simulink model "Final_Project"  (R2021b)
settings: Solver=VariableStepAuto  StartTime=0.0  StopTime=10.0  RelTol=1e-3
undefined symbols (not defined in the file or in its folder): A, Aobs, B, Bobs, C, Cobs, Cobs1, Continuous, D, Dobs, K, N2, r0, Time
libraries: ctrlSharedLib x1, slpidlib x1
settings Model: Creator=AzamaoZ  LastModifiedBy=AzamaoZ
settings DataIOCC: ExternalInput=getinputstruct(op_trim1)  InitialState=getstatestruct(op_trim1)  LoadExternalInput=on  LoadInitialState=on

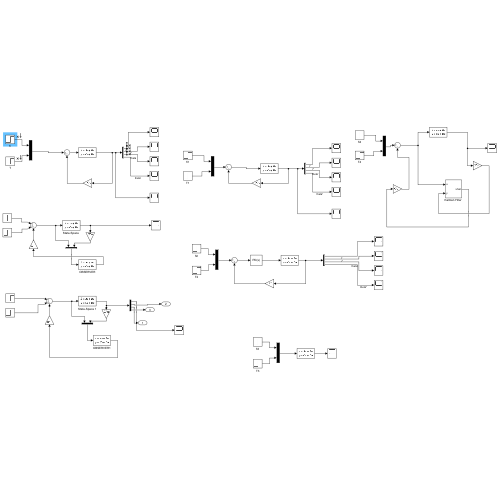
[thumbnail: Simulink's stored preview of the top-level diagram]
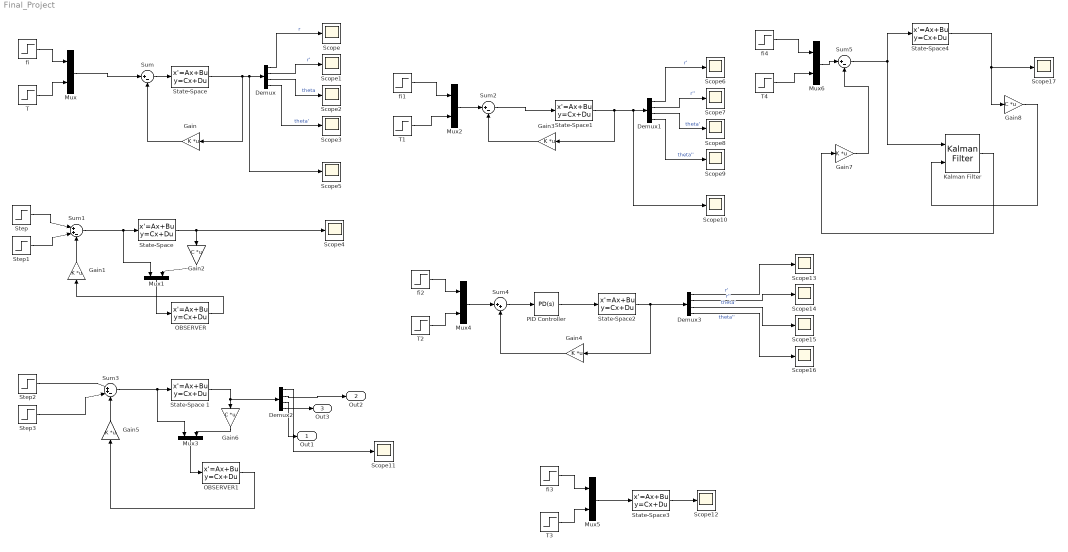
== system Final_Project ==
  Demux{,1..3} (4 alike) : Demux
  Gain{,1,3..5,7} (6 alike) : Gain  Gain=K  Multiplication=Matrix(K*u)
  Gain2 : Gain  Gain=C  Multiplication=Matrix(K*u)
  Gain6 : Gain  Gain=C  Multiplication=Matrix(K*u)
  Gain8 : Gain  Gain=C  Multiplication=Matrix(K*u)
  "Kalman Filter " : ctrlSharedLib/Kalman Filter  TimeDomain=Continuous-Time  UseCurrentEstimator=on  ModelSource=Individual A, B, C, D matrices  ModelSourceVariable=ss(0.95,1,1,0,1)  A=A  B=B  C=C  D=D  NumberOfStates=1  NumberOfInputs=1  NumberOfOutputs=1  InitialEstimateSource=Dialog  X0=10  P0=10  UseK=off  UseGH=off  NumberOfProcessNoiseInputs=1  G=1  TimeInvariantG=on  H=0  TimeInvariantH=on  Q=Q2  TimeInvariantQ=on  R=200  TimeInvariantR=on  N=N2  TimeInvariantN=on  AddInputPort=on  AddEnablePort=off  OutputEstimatedY=off  OutputP=off  Ts=-1
  Mux{,1..6} (7 alike) : Mux  Inputs=2
  OBSERVER : StateSpace  A=Aobs  B=Bobs  C=C  D=Dobs  InitialCondition=0
  OBSERVER1 : StateSpace  A=Aobs  B=Bobs  C=Cobs  D=Dobs  InitialCondition=0
  PID Controller : slpidlib/PID Controller  Controller=PD  Form=Parallel  TimeDomain=Continuous-time  UseExternalTs=off  SampleTime=-1  IntegratorMethod=Forward Euler  FilterMethod=Forward Euler  ControllerParametersSource=internal  P=0.02  I=1  D=0.01  UseFilter=on  N=100  TunerSelectOption=Frequency Response Based  InitialConditionSource=internal  InitialConditionForIntegrator=0  InitialConditionForFilter=0  DifferentiatorICPrevScaledInput=0  ExternalReset=none  TrackingMode=off  Kt=1  LimitOutput=off  SatLimitsSource=internal  UpperSaturationLimit=inf  LowerSaturationLimit=-inf  LinearizeAsGain=on  AntiWindupMode=none  Kb=1  POutMin=[]  POutMax=[]  IOutMin=[]  IOutMax=[]  DOutMin=[]  DOutMax=[]  NOutMin=[]  NOutMax=[]  SumOutMin=[]  SumOutMax=[]  SaturationOutMin=[]  SaturationOutMax=[]  PParamMin=[]  PParamMax=[]  IParamMin=[]  IParamMax=[]  DParamMin=[]  DParamMax=[]  NParamMin=[]  NParamMax=[]  KbParamMin=[]  KbParamMax=[]  KtParamMin=[]  KtParamMax=[]  KbOutMin=[]  KbOutMax=[]  KtOutMin=[]  KtOutMax=[]  IntegratorOutMin=[]  IntegratorOutMax=[]  FilterOutMin=[]  FilterOutMax=[]  SumI1OutMin=[]  SumI1OutMax=[]  SumI2OutMin=[]  SumI2OutMax=[]  SumI3OutMin=[]  SumI3OutMax=[]  SumI4OutMin=[]  SumI4OutMax=[]  SumDOutMin=[]  SumDOutMax=[]  DifferentiatorOutMin=[]  DifferentiatorOutMax=[]  FilterDiffOutCoefMin=[]  FilterDiffOutCoefMax=[]  ReciprocalOutMin=[]  ReciprocalOutMax=[]  SumDenOutMin=[]  SumDenOutMax=[]  SumNumOutMin=[]  SumNumOutMax=[]  DivideOutMin=[]  DivideOutMax=[]  UdiffTsProdOutMin=[]  UdiffTsProdOutMax=[]  NTsProdOutMin=[]  NTsProdOutMax=[]  UintegralTsProdOutMin=[]  UintegralTsProdOutMax=[]  UngainTsProdOutMin=[]  UngainTsProdOutMax=[]  IntegratorContinuousStateAttributes=''  IntegratorStateMustResolveToSignalObject=off  IntegratorRTWStateStorageClass=Auto  FilterContinuousStateAttributes='radius'  FilterStateMustResolveToSignalObject=off  FilterRTWStateStorageClass=Auto  ParallelPVariant=InternalParameters  IdealPVariant=Disabled  IVariant=Disabled  DVariant=InternalParameters  IntegratorVariant=Disabled  SatVariant=Disabled  AWVariant=Disabled  PCopyVariant=Disabled  TRVariant=Disabled  FdbkBlocksVariant=Forward  IdealPFdbkVariant=Disabled  SatFdbkVariant=Disabled  DerivativeFilterVariant=ContFilter  NVariant=InternalParameters  NCopyVariant=Disabled  FilterICVariant=InternalICsFilter  IntegratorICVariant=Disabled  ExternalResetVariant=Disabled  TRSumVariant=Passthrough  SumFdbkVariant=Disabled  SumVariant=Sum_PD  TsampFilterVariant=InternalTs  TsampNgainVariant=Passthrough  TsampIntegralVariant=Disabled_SignalSpec  ExternalSaturationOutDataTypeStr=Inherit: Same as second input
  Scope{,1..17} (18 alike) : Scope
  State-Space{,2..4} (4 alike) : StateSpace  A=A  B=B  C=C  D=D  InitialCondition=0
  "State-Space " : StateSpace  A=A  B=B  C=C  D=D  InitialCondition=0
  State-Space 1 : StateSpace  A=A  B=B  C=C  D=D  InitialCondition=0
  State-Space1 : StateSpace  A=A  B=B  C=Cobs1  D=D  InitialCondition=0
  Step : Step  Time=0  SampleTime=0
  Step1 : Step  Time=0  SampleTime=0
  Step2 : Step  SampleTime=0
  Step3 : Step  SampleTime=0
  Sum : Sum  Inputs=|+-
  Sum1 : Sum  Inputs=|++-
  Sum2 : Sum  Inputs=|+-
  Sum3 : Sum  Inputs=|++-
  Sum4 : Sum  Inputs=|++
  Sum5 : Sum  Inputs=|+-
  T{,1,3..4} (4 alike) : Step  Time=0  SampleTime=0
  T2 : Step  Time=0  Before=r0  After=r0*1.1  SampleTime=0
  fi{,1,3..4} (4 alike) : Step  Time=0  SampleTime=0
  fi2 : Step  Time=0  Before=r0  After=r0*1.1  SampleTime=0
  Out1 : Outport
  Out2 : Outport  Port=2
  Out3 : Outport  Port=3
  wires:
  Demux1/1 -> Scope6/1  "r'"
  T1/1 -> Mux2/2
  Demux1/4 -> Scope9/1  "theta''"
  Demux1/3 -> Scope8/1  "theta'"
  Demux1/2 -> Scope7/1  "r''"
  fi1/1 -> Mux2/1
  Demux2/4 -> Out3/1
  Demux2/2 -> Out2/1
  OBSERVER1/1 -> Gain5/1
  Step3/1 -> Sum3/2
  Gain6/1 -> Mux3/2
  Step2/1 -> Sum3/1
  State-Space 1/1 -> Demux2/1, Gain6/1
  Mux3/1 -> OBSERVER1/1
  Gain5/1 -> Sum3/3
  Sum3/1 -> Mux3/1, State-Space 1/1
  Gain1/1 -> Sum1/3
  Step/1 -> Sum1/1
  Gain2/1 -> Mux1/2
  Mux1/1 -> OBSERVER/1
  "State-Space "/1 -> Scope4/1, Gain2/1
  Sum1/1 -> Mux1/1, "State-Space "/1
  OBSERVER/1 -> Gain1/1
  Step1/1 -> Sum1/2
  T/1 -> Mux/2
  State-Space/1 -> Gain/1, Scope5/1, Demux/1
  Mux/1 -> Sum/1
  Demux/3 -> Scope2/1  "theta"
  Sum/1 -> State-Space/1
  Demux/4 -> Scope3/1  "theta'"
  Demux/2 -> Scope1/1  "r'"
  Gain/1 -> Sum/2
  fi/1 -> Mux/1
  fi2/1 -> Mux4/1
  T2/1 -> Mux4/2
  Mux4/1 -> Sum4/1
  Demux3/2 -> Scope14/1  "r''"
  Demux3/4 -> Scope16/1  "theta''"
  Demux3/3 -> Scope15/1  "theta'"
  State-Space2/1 -> Demux3/1, Gain4/1
  Demux3/1 -> Scope13/1  "r'"
  Demux/1 -> Scope/1  "r"
  PID Controller/1 -> State-Space2/1
  Sum4/1 -> PID Controller/1
  State-Space1/1 -> Gain3/1, Scope10/1, Demux1/1
  Gain3/1 -> Sum2/2
  Sum2/1 -> State-Space1/1
  Mux2/1 -> Sum2/1
  fi3/1 -> Mux5/1
  Mux5/1 -> State-Space3/1
  T3/1 -> Mux5/2
  State-Space3/1 -> Scope12/1
  Demux2/3 -> Out1/1
  Demux2/1 -> Scope11/1
  Gain4/1 -> Sum4/2
  "Kalman Filter "/1 -> Gain7/1
  Gain8/1 -> "Kalman Filter "/2
  Sum5/1 -> "Kalman Filter "/1, State-Space4/1
  Gain7/1 -> Sum5/2
  State-Space4/1 -> Scope17/1, Gain8/1
  Mux6/1 -> Sum5/1
  fi4/1 -> Mux6/1
  T4/1 -> Mux6/2
